simulink model "M10B39"  (R2025a)
settings: Solver=ode23tb  StartTime=0.0  StopTime=20  FixedStep=0.001  MaxStep=0.01  RelTol=1e-3  EnableMultiTasking=on
InitFcn:
  | initAll
values from neighbouring files (symbols this model uses):
  acom = 100    [initAll.m]    (also in initAll_V2.m)
  bcom = 50    [initAll.m]    (also in initAll_V2.m)
  commun = 0*commun    [initAll.m]    (also in initAll_V2.m)
  DataDelay = 0.0*DataDelay    [initAll.m]    (also in initAll_V2.m)
  fB = 50    [initAll.m]    (also in initAll_V2.m)
  Geninit = Generator_init(opdata,SynMach_in_gidx)    [initAll.m]    (also in initAll_V2.m)
  lam = 100    [initAll.m]    (also in initAll_V2.m)
  SgridB = 100    [initAll.m]    (also in initAll_V2.m)
  wB = 2*pi*fB    (= 314.159265359)    [initAll.m]    (also in initAll_V2.m)
undefined symbols (not defined in the file or in its folder): AVm0, c1, c2, c3, c4, c5, c6, cp_nom, ESinit, lambda_nom, P_wind_base, Pelec_base, Pnom, Windinit, YY_load
libraries: spsBistableLib x10, simulink_extras x6, simulink x1
(part 3 of 8)

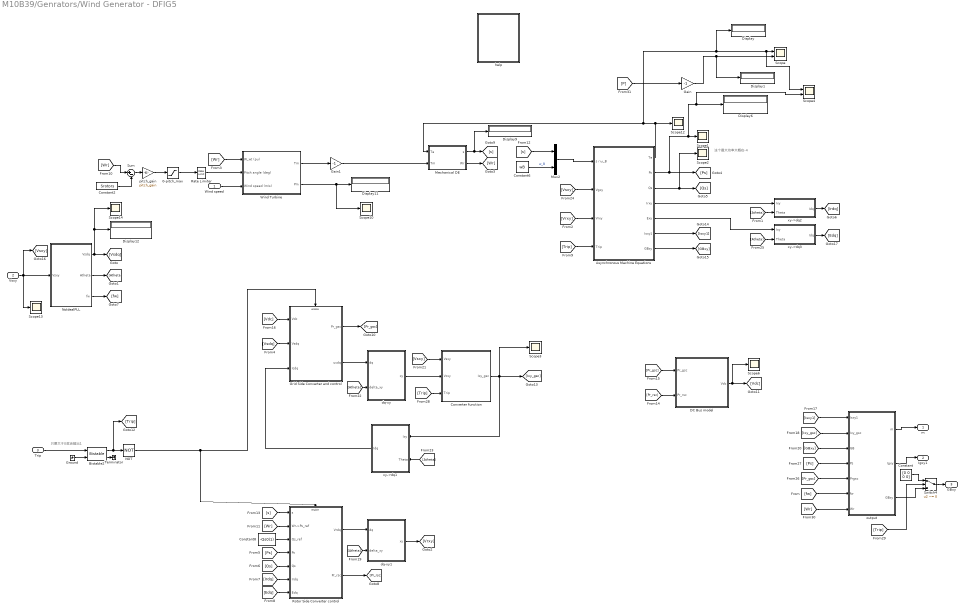
== system M10B39/Genrators/Wind Generator - DFIG5 ==
  note: 只要大于0就会输出1
  note: 这个最大功率大概在-4
  Wind speed : Inport
  Vsxy : Inport  Port=2
  Trip : Inport  Port=3
  0-pitch_max : Saturate  UpperLimit=pitch_max  LowerLimit=0
  "Asynchronous Machine Equations " : Subsystem
  Bistable2 : spsBistableLib/Bistable  Qpriority=Set  ic=0  Ts=0
  Constant : Constant  Value=[0 0 0 0]
  Constant2 : Constant  Value=Srotors
  Constant6 : Constant  Value=wB
  Constant8 : Constant  Value=-Qs0(1)
  Converter function : Subsystem
  DC Bus model : Subsystem
  Display{,1,6,9,11..12} (6 alike) : Display
  Gain : Gain  Gain=-1
  Gain1 : Gain  Gain=-1
  Grid Side Converter and control : Subsystem
  Ground : Ground
  Mechanical DE : Subsystem
  Mux2 : Mux  Inputs=2
  NOT : Logic  Operator=NOT  AllPortsSameDT=off  OutDataTypeStr=boolean
  NoIdealPLL : Subsystem  VariantControl=Noideal_PLL_Wind1
  "Rate Limiter   " : RateLimiter  RisingSlewLimit=pitch_rate  FallingSlewLimit=-pitch_rate
  Rotor Side Converter control : Subsystem
  Scope : Scope  NumInputPorts=2
      settings: ActiveDisplayYMinimum=-1.1471  ActiveDisplayYMaximum=-0.81376
  Scope{1..3,6,10,12..14} (8 alike) : Scope
      Scope1 settings: ActiveDisplayYMinimum=-2.187000000000014  ActiveDisplayYMaximum=-2.186999999999987  DataLoggingVariableName=ScopeData2
      Scope10 settings: ActiveDisplayYMinimum=0.84538  ActiveDisplayYMaximum=0.84729
      Scope12 settings: ActiveDisplayYMinimum=-1.99497  ActiveDisplayYMaximum=-0.90484  DataLoggingVariableName=ScopeData6
      Scope13 settings: ActiveDisplayYMinimum=-1.25875  ActiveDisplayYMaximum=1.25908  DataLoggingVariableName=ScopeData2
      Scope14 settings: ActiveDisplayYMinimum=1.003489  ActiveDisplayYMaximum=1.0035  DataLoggingVariableName=ScopeData3
      Scope2 settings: ActiveDisplayYMinimum=-0.00085  ActiveDisplayYMaximum=0.00099  DataLoggingVariableName=ScopeData2
      Scope3 settings: ActiveDisplayYMinimum=-0.01172  ActiveDisplayYMaximum=0.10551
      Scope6 settings: ActiveDisplayYMinimum=2.82799999999992  ActiveDisplayYMaximum=2.82800000000004  DataLoggingVariableName=ScopeData5
  Scope4 : Scope  NumInputPorts=2
      settings: ActiveDisplayYMinimum=-1.13533  ActiveDisplayYMaximum=-0.91965  DataLoggingVariableName=ScopeData2
  Sum : Sum  Inputs=|+-  SaturateOnIntegerOverflow=on
  Switch4 : Switch  Criteria=u2 ~= 0  Threshold=0.5  InputSameDT=off
  Terminator : Terminator
  Wind Turbine : Subsystem
  dq-xy : Subsystem
  dq-xy1 : Subsystem
  help : Subsystem
  output : Subsystem
  pitch_gain : Gain  Gain=pitch_gain  SaturateOnIntegerOverflow=on  OutDataTypeStr=Inherit: Same as input  ParamDataTypeStr=Inherit: Same as input
  xy->dq1 : Subsystem
  xy->dq2 : Subsystem
  xy->dq3 : Subsystem
  m : Outport
  Igxy1 : Outport  Port=2
  GBxy : Outport  Port=3
  wires:
  [Wr] -> output/7(Wr)
  Gain1/1 -> Mechanical DE/2(Tm)
  output/3(GBxy) -> Switch4/3
  Switch4/1 -> GBxy/1
  Constant/1 -> Switch4/1
  [Trip] -> Switch4/2
  [Trip] -> Converter function/3(Trip)
  [Trip] -> "Asynchronous Machine Equations "/4("Trip ")
  [Wr] -> Sum/1
  0-pitch_max/1 -> "Rate Limiter   "/1
  pitch_gain/1 -> 0-pitch_max/1
  Constant2/1 -> Sum/2
  Sum/1 -> pitch_gain/1
  NOT/1 -> Rotor Side Converter control/Enable, Grid Side Converter and control/Enable
  Trip/1 -> Bistable2/1
  Bistable2/2 -> Terminator/1
  Bistable2/1 -> NOT/1, [Trip]
  Ground/1 -> Bistable2/2
  [fw] -> output/6(fw)
  [Pr_gsc] -> output/5(Prgsc)
  [Ps] -> output/4(Ps)
  output/1(m) -> m/1
  [Isxy1] -> output/1(Isxy1)
  [Ixy_gsc] -> output/2(Ixy_gsc)
  output/2(Igxy) -> Igxy1/1
  xy->dq3/1(Idq) -> [Edq]
  [Atheta] -> xy->dq3/2(Theta)
  xy->dq2/1(Idq) -> [Irdq]
  [Atheta] -> xy->dq2/2(Theta)
  dq-xy1/1(xy) -> [Vrxy]
  [Atheta] -> dq-xy1/2(delta_xy)
  xy->dq1/1(Idq) -> Grid Side Converter and control/3(Icdq)
  [Atheta] -> xy->dq1/2(Theta)
  [Atheta] -> dq-xy/2(delta_xy)
  dq-xy/1(xy) -> Converter function/2(Vcxy)
  Grid Side Converter and control/2(ucdq) -> dq-xy/1(dq)
  [Vsxy] -> Converter function/1(Vsxy)
  NoIdealPLL/3(fw) -> [fw]
  Vsxy/1 -> [Vsxy], Scope13/1, NoIdealPLL/1(Vsxy)
  [GBxy] -> output/3(GB)
  [Pr_rsc] -> DC Bus model/2(Pr_rsc)
  "Asynchronous Machine Equations "/1(Te) -> Scope12/1, Display/1, Scope4/1, Scope/1, Mechanical DE/1(Te)
  Constant8/1 -> Rotor Side Converter control/3(Qs_ref)
  [Wr] -> Wind Turbine/1(W_wt (pu))
  "Asynchronous Machine Equations "/4(Irxy) -> xy->dq2/1(Ixy)
  Converter function/1(Ixy_gsc) -> [Ixy_gsc], xy->dq1/1(Ixy), Scope3/1
  [Vrxy] -> "Asynchronous Machine Equations "/3(Vrxy)
  "Asynchronous Machine Equations "/6(Isxy1) -> [Isxy1]
  [Qs] -> Rotor Side Converter control/5(Qs)
  [Vdc] -> Grid Side Converter and control/1(Vdc)
  [Pr_gsc] -> DC Bus model/1(Pr_gsc)
  "Asynchronous Machine Equations "/2(Ps) -> Scope1/1, Scope4/2, Display6/1, [Ps]
  Mechanical DE/1("s ") -> [s], Display9/1
  [s] -> Mux2/1
  [Vsdq] -> Grid Side Converter and control/2(Vsdq)
  Grid Side Converter and control/1(Pr_gsc) -> [Pr_gsc]
  NoIdealPLL/2(Atheta) -> [Atheta]
  DC Bus model/1(Vdc) -> [Vdc], Scope6/1
  [Vsxy] -> "Asynchronous Machine Equations "/2(Vgxy)
  Wind Turbine/1(Tm) -> Gain1/1
  [Irdq] -> Rotor Side Converter control/6(Irdq)
  Mux2/1 -> "Asynchronous Machine Equations "/1(s / ω_B)
  "Asynchronous Machine Equations "/7(GBxy) -> [GBxy]
  "Rate Limiter   "/1 -> Wind Turbine/2(Pitch angle (deg))
  NoIdealPLL/1(Vsdq) -> Display12/1, Scope14/1, [Vsdq]
  [s] -> Rotor Side Converter control/1(s)
  Rotor Side Converter control/2(Pr_rsc) -> [Pr_rsc]
  Mechanical DE/2(Wr) -> [Wr]
  [Wr] -> Rotor Side Converter control/2(Wr->Ps_ref)
  Wind Turbine/2(Pm) -> Display11/1, Scope10/1
  "Asynchronous Machine Equations "/3(Qs) -> [Qs], Scope2/1
  Wind speed/1 -> Wind Turbine/3(Wind speed (m/s))
  [Ps] -> Rotor Side Converter control/4(Ps)
  Rotor Side Converter control/1(Vrdq) -> dq-xy1/1(dq)
  [Edq] -> Rotor Side Converter control/7(Edq)
  Constant6/1 -> Mux2/2  "w_B"
  "Asynchronous Machine Equations "/5(Exy) -> xy->dq3/1(Ixy)
  [P] -> Gain/1
  Gain/1 -> Display1/1, Scope/2

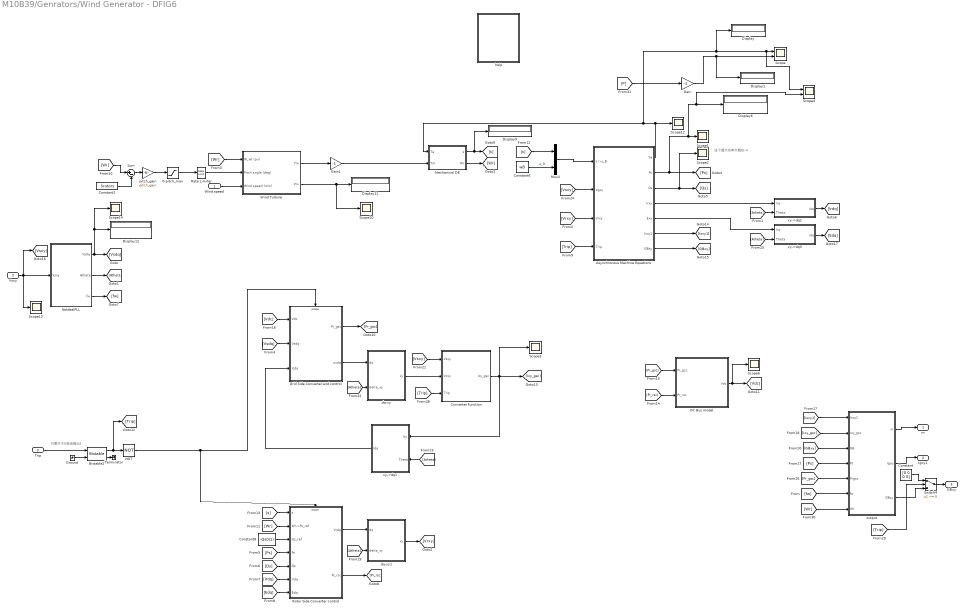
== system M10B39/Genrators/Wind Generator - DFIG6 ==
  note: 只要大于0就会输出1
  note: 这个最大功率大概在-4
  Wind speed : Inport
  Vsxy : Inport  Port=2
  Trip : Inport  Port=3
  0-pitch_max : Saturate  UpperLimit=pitch_max  LowerLimit=0
  "Asynchronous Machine Equations " : Subsystem
  Bistable2 : spsBistableLib/Bistable  Qpriority=Set  ic=0  Ts=0
  Constant : Constant  Value=[0 0 0 0]
  Constant2 : Constant  Value=Srotors
  Constant6 : Constant  Value=wB
  Constant8 : Constant  Value=-Qs0(1)
  Converter function : Subsystem
  DC Bus model : Subsystem
  Display{,1,6,9,11..12} (6 alike) : Display
  Gain : Gain  Gain=-1
  Gain1 : Gain  Gain=-1
  Grid Side Converter and control : Subsystem
  Ground : Ground
  Mechanical DE : Subsystem
  Mux2 : Mux  Inputs=2
  NOT : Logic  Operator=NOT  AllPortsSameDT=off  OutDataTypeStr=boolean
  NoIdealPLL : Subsystem  VariantControl=Noideal_PLL_Wind1
  "Rate Limiter   " : RateLimiter  RisingSlewLimit=pitch_rate  FallingSlewLimit=-pitch_rate
  Rotor Side Converter control : Subsystem
  Scope : Scope  NumInputPorts=2
      settings: ActiveDisplayYMinimum=-1.1471  ActiveDisplayYMaximum=-0.81376
  Scope{1..3,6,10,12..14} (8 alike) : Scope
      Scope1 settings: ActiveDisplayYMinimum=-2.187000000000014  ActiveDisplayYMaximum=-2.186999999999987  DataLoggingVariableName=ScopeData2
      Scope10 settings: ActiveDisplayYMinimum=0.84538  ActiveDisplayYMaximum=0.84729
      Scope12 settings: ActiveDisplayYMinimum=-1.99497  ActiveDisplayYMaximum=-0.90484  DataLoggingVariableName=ScopeData6
      Scope13 settings: ActiveDisplayYMinimum=-1.25875  ActiveDisplayYMaximum=1.25908  DataLoggingVariableName=ScopeData2
      Scope14 settings: ActiveDisplayYMinimum=1.003489  ActiveDisplayYMaximum=1.0035  DataLoggingVariableName=ScopeData3
      Scope2 settings: ActiveDisplayYMinimum=-0.00085  ActiveDisplayYMaximum=0.00099  DataLoggingVariableName=ScopeData2
      Scope3 settings: ActiveDisplayYMinimum=-0.01172  ActiveDisplayYMaximum=0.10551
      Scope6 settings: ActiveDisplayYMinimum=2.82799999999992  ActiveDisplayYMaximum=2.82800000000004  DataLoggingVariableName=ScopeData5
  Scope4 : Scope  NumInputPorts=2
      settings: ActiveDisplayYMinimum=-1.13533  ActiveDisplayYMaximum=-0.91965  DataLoggingVariableName=ScopeData2
  Sum : Sum  Inputs=|+-  SaturateOnIntegerOverflow=on
  Switch4 : Switch  Criteria=u2 ~= 0  Threshold=0.5  InputSameDT=off
  Terminator : Terminator
  Wind Turbine : Subsystem
  dq-xy : Subsystem
  dq-xy1 : Subsystem
  help : Subsystem
  output : Subsystem
  pitch_gain : Gain  Gain=pitch_gain  SaturateOnIntegerOverflow=on  OutDataTypeStr=Inherit: Same as input  ParamDataTypeStr=Inherit: Same as input
  xy->dq1 : Subsystem
  xy->dq2 : Subsystem
  xy->dq3 : Subsystem
  m : Outport
  Igxy1 : Outport  Port=2
  GBxy : Outport  Port=3
  wires:
  [Wr] -> output/7(Wr)
  Gain1/1 -> Mechanical DE/2(Tm)
  output/3(GBxy) -> Switch4/3
  Switch4/1 -> GBxy/1
  Constant/1 -> Switch4/1
  [Trip] -> Switch4/2
  [Trip] -> Converter function/3(Trip)
  [Trip] -> "Asynchronous Machine Equations "/4("Trip ")
  [Wr] -> Sum/1
  0-pitch_max/1 -> "Rate Limiter   "/1
  pitch_gain/1 -> 0-pitch_max/1
  Constant2/1 -> Sum/2
  Sum/1 -> pitch_gain/1
  NOT/1 -> Rotor Side Converter control/Enable, Grid Side Converter and control/Enable
  Trip/1 -> Bistable2/1
  Bistable2/2 -> Terminator/1
  Bistable2/1 -> NOT/1, [Trip]
  Ground/1 -> Bistable2/2
  [fw] -> output/6(fw)
  [Pr_gsc] -> output/5(Prgsc)
  [Ps] -> output/4(Ps)
  output/1(m) -> m/1
  [Isxy1] -> output/1(Isxy1)
  [Ixy_gsc] -> output/2(Ixy_gsc)
  output/2(Igxy) -> Igxy1/1
  xy->dq3/1(Idq) -> [Edq]
  [Atheta] -> xy->dq3/2(Theta)
  xy->dq2/1(Idq) -> [Irdq]
  [Atheta] -> xy->dq2/2(Theta)
  dq-xy1/1(xy) -> [Vrxy]
  [Atheta] -> dq-xy1/2(delta_xy)
  xy->dq1/1(Idq) -> Grid Side Converter and control/3(Icdq)
  [Atheta] -> xy->dq1/2(Theta)
  [Atheta] -> dq-xy/2(delta_xy)
  dq-xy/1(xy) -> Converter function/2(Vcxy)
  Grid Side Converter and control/2(ucdq) -> dq-xy/1(dq)
  [Vsxy] -> Converter function/1(Vsxy)
  NoIdealPLL/3(fw) -> [fw]
  Vsxy/1 -> [Vsxy], Scope13/1, NoIdealPLL/1(Vsxy)
  [GBxy] -> output/3(GB)
  [Pr_rsc] -> DC Bus model/2(Pr_rsc)
  "Asynchronous Machine Equations "/1(Te) -> Scope12/1, Display/1, Scope4/1, Scope/1, Mechanical DE/1(Te)
  Constant8/1 -> Rotor Side Converter control/3(Qs_ref)
  [Wr] -> Wind Turbine/1(W_wt (pu))
  "Asynchronous Machine Equations "/4(Irxy) -> xy->dq2/1(Ixy)
  Converter function/1(Ixy_gsc) -> [Ixy_gsc], xy->dq1/1(Ixy), Scope3/1
  [Vrxy] -> "Asynchronous Machine Equations "/3(Vrxy)
  "Asynchronous Machine Equations "/6(Isxy1) -> [Isxy1]
  [Qs] -> Rotor Side Converter control/5(Qs)
  [Vdc] -> Grid Side Converter and control/1(Vdc)
  [Pr_gsc] -> DC Bus model/1(Pr_gsc)
  "Asynchronous Machine Equations "/2(Ps) -> Scope1/1, Scope4/2, Display6/1, [Ps]
  Mechanical DE/1("s ") -> [s], Display9/1
  [s] -> Mux2/1
  [Vsdq] -> Grid Side Converter and control/2(Vsdq)
  Grid Side Converter and control/1(Pr_gsc) -> [Pr_gsc]
  NoIdealPLL/2(Atheta) -> [Atheta]
  DC Bus model/1(Vdc) -> [Vdc], Scope6/1
  [Vsxy] -> "Asynchronous Machine Equations "/2(Vgxy)
  Wind Turbine/1(Tm) -> Gain1/1
  [Irdq] -> Rotor Side Converter control/6(Irdq)
  Mux2/1 -> "Asynchronous Machine Equations "/1(s / ω_B)
  "Asynchronous Machine Equations "/7(GBxy) -> [GBxy]
  "Rate Limiter   "/1 -> Wind Turbine/2(Pitch angle (deg))
  NoIdealPLL/1(Vsdq) -> Display12/1, Scope14/1, [Vsdq]
  [s] -> Rotor Side Converter control/1(s)
  Rotor Side Converter control/2(Pr_rsc) -> [Pr_rsc]
  Mechanical DE/2(Wr) -> [Wr]
  [Wr] -> Rotor Side Converter control/2(Wr->Ps_ref)
  Wind Turbine/2(Pm) -> Display11/1, Scope10/1
  "Asynchronous Machine Equations "/3(Qs) -> [Qs], Scope2/1
  Wind speed/1 -> Wind Turbine/3(Wind speed (m/s))
  [Ps] -> Rotor Side Converter control/4(Ps)
  Rotor Side Converter control/1(Vrdq) -> dq-xy1/1(dq)
  [Edq] -> Rotor Side Converter control/7(Edq)
  Constant6/1 -> Mux2/2  "w_B"
  "Asynchronous Machine Equations "/5(Exy) -> xy->dq3/1(Ixy)
  [P] -> Gain/1
  Gain/1 -> Display1/1, Scope/2

== system M10B39/Genrators/ES1/ control1 ==
  usdq : Inport
  isdq : Inport  Port=2
  delta : Inport  Port=3
  Enable : EnablePort
  Add : Sum  Inputs=|-+
  Add2 : Sum  Inputs=|-+
  Add3 : Sum
  Add4 : Sum  Inputs=-+
  Add6 : Sum  Inputs=|++
  Add7 : Sum  Inputs=+-
  Complex to Magnitude-Angle : ComplexToMagnitudeAngle
  Complex to Real-Imag1 : ComplexToRealImag
  Constant : Constant
  Constant1 : Constant  Value=usd0
  Constant2 : Constant  Value=0
  Constant3 : Constant  Value=Q0
  Constant4 : Constant
  Demux : Demux  Outputs=2
  Demux1 : Demux  Outputs=2
  Gain : Gain  Gain=0.01
  Gain1 : Gain  Gain=-1
  K5 : Gain  Gain=Lpr  SaturateOnIntegerOverflow=on  OutDataTypeStr=Inherit: Same as input  ParamDataTypeStr=Inherit: Same as input
  K6 : Gain  Gain=Lpr  SaturateOnIntegerOverflow=on  OutDataTypeStr=Inherit: Same as input  ParamDataTypeStr=Inherit: Same as input
  Magnitude-Angle to Complex : MagnitudeAngleToComplex
  Product{1,4..6} (4 alike) : Product  RndMeth=Zero
  Real-Imag to Complex : RealImagToComplex
  Scope : Scope
      settings: ActiveDisplayYMinimum=-1.90229  ActiveDisplayYMaximum=-1.00495  DataLoggingVariableName=ScopeData6
  Scope1 : Scope
      settings: ActiveDisplayYMinimum=1.01143  ActiveDisplayYMaximum=1.18506  DataLoggingVariableName=ScopeData8
  Scope2 : Scope  NumInputPorts=2
      settings: ActiveDisplayYMinimum=-1E-15  ActiveDisplayYMaximum=1.3E-14  DataLoggingVariableName=ScopeData9
  Scope3 : Scope  NumInputPorts=2
      settings: ActiveDisplayYMinimum=-0.06902  ActiveDisplayYMaximum=1.69489  DataLoggingVariableName=ScopeData4
  Scope7 : Scope  NumInputPorts=2
      settings: ActiveDisplayYMinimum=-1.01296  ActiveDisplayYMaximum=-0.62415
  Sum : Sum  Inputs=|+-
  Sum2 : Sum  Inputs=|+-  SaturateOnIntegerOverflow=on
  Sum23 : Sum  Inputs=|+-  SaturateOnIntegerOverflow=on
  Sum9 : Sum  Inputs=|+-  SaturateOnIntegerOverflow=on
  control_AC_voltage : Subsystem  VariantControl=VSC1q_Variant2
  control_AC_voltage1 : Subsystem  VariantControl=VSC1q_Variant2
  in_D_PI : Subsystem  mask{KP_=KpId_VSC_A, KI_=KiId_VSC_A, Upper_limit=inf, Lower_limit=-inf, Upper_saturation_limit=inf, Lower_saturation_limit=-inf, integrator_init=Md_A_0}
      mask prompts: KP_ "比例系数P"; KI_ "积分系数I"; Upper_limit "限幅上限"; Lower_limit "限幅下限"; Upper_saturation_limit "积分饱和上限"; Lower_saturation_limit "积分饱和下限"; integrator_init "积分初始值"
      mask DialogControl Container4 Prompt: 控制参数
      mask DialogControl Container5 Prompt: 初始值
      mask Display: disp('PI')
  in_Q_PI : Subsystem  mask{KP_=KpIq_VSC_A, KI_=KiIq_VSC_A, Upper_limit=inf, Lower_limit=-inf, Upper_saturation_limit=inf, Lower_saturation_limit=-inf, integrator_init=Mq_A_0}
      mask prompts: KP_ "比例系数P"; KI_ "积分系数I"; Upper_limit "限幅上限"; Lower_limit "限幅下限"; Upper_saturation_limit "积分饱和上限"; Lower_saturation_limit "积分饱和下限"; integrator_init "积分初始值"
      mask DialogControl Container4 Prompt: 控制参数
      mask DialogControl Container5 Prompt: 初始值
      mask Display: disp('PI')
  ucx : Outport
  ucy : Outport  Port=2
  wires:
  Magnitude-Angle to Complex/1 -> Complex to Real-Imag1/1
  Add/1 -> Real-Imag to Complex/2
  Add2/1 -> Real-Imag to Complex/1
  delta/1 -> Add6/2
  Add6/1 -> Magnitude-Angle to Complex/2
  Complex to Magnitude-Angle/2 -> Add6/1
  Sum9/1 -> in_D_PI/1(In1)
  K5/1 -> Add3/1
  [usd] -> Add3/2
  Add3/1 -> Add2/2
  in_D_PI/1(Out1) -> Add2/1
  Constant/1 -> Product4/2
  [isq] -> Product4/1
  [isd] -> Scope7/2, Sum9/2
  Product4/1 -> K5/1
  Demux1/1 -> [isd]
  Demux/1 -> [usd]
  Demux1/2 -> [isq]
  Demux/2 -> [usq]
  isdq/1 -> Demux1/1
  usdq/1 -> Demux/1
  [usq] -> Add4/2
  K6/1 -> Add4/1
  in_Q_PI/1(Out1) -> Add/1
  Sum23/1 -> in_Q_PI/1(In1)
  [isd] -> Product1/1
  [isq] -> Sum23/2, Scope3/2
  Product1/1 -> K6/1
  Constant4/1 -> Product1/2
  Add4/1 -> Add/2
  Real-Imag to Complex/1 -> Complex to Magnitude-Angle/1
  Complex to Magnitude-Angle/1 -> Magnitude-Angle to Complex/1
  Complex to Real-Imag1/1 -> ucx/1
  Complex to Real-Imag1/2 -> ucy/1
  [usd] -> Scope1/1, control_AC_voltage/1(usd)
  control_AC_voltage/1(isdref) -> Scope7/1, Sum9/1
  [isq] -> Product5/2
  Product5/1 -> Add7/2
  [usd] -> Product5/1
  [isd] -> Product6/2
  Product6/1 -> Add7/1
  [usq] -> Product6/1
  Gain/1 -> Sum/2
  control_AC_voltage1/1(isqref) -> Scope3/1, Sum23/1
  [usq] -> Scope2/1, control_AC_voltage1/1(usq)
  Constant2/1 -> Scope2/2, control_AC_voltage1/2(usqref)
  Add7/1 -> Scope/1, Gain1/1
  Sum2/1 -> Gain/1
  Constant3/1 -> Sum2/2
  Gain1/1 -> Sum2/1
  Sum/1 -> control_AC_voltage/2(usdref)
  Constant1/1 -> Sum/1

== system M10B39/Genrators/ES1/in_D_PI ==
  In1 : Inport
  Ki : Gain  Gain=KI_  SaturateOnIntegerOverflow=on  OutDataTypeStr=Inherit: Same as input  ParamDataTypeStr=Inherit: Same as input
  Kp : Gain  Gain=KP_  SaturateOnIntegerOverflow=on  OutDataTypeStr=Inherit: Same as input  ParamDataTypeStr=Inherit: Same as input
  Saturation2 : Saturate  UpperLimit=Upper_limit  LowerLimit=Lower_limit
  Sum12 : Sum  SaturateOnIntegerOverflow=on
  integrator : Integrator  InitialCondition=integrator_init  LimitOutput=on  UpperSaturationLimit=Upper_saturation_limit  LowerSaturationLimit=Lower_saturation_limit
  Out1 : Outport
  wires:
  In1/1 -> Ki/1, Kp/1
  Kp/1 -> Sum12/2
  Ki/1 -> integrator/1
  integrator/1 -> Sum12/1
  Saturation2/1 -> Out1/1
  Sum12/1 -> Saturation2/1

== system M10B39/Genrators/ES1/output ==
  is_xy : Inport
  Pe : Inport  Port=2
  Brecx : Constant  Value=0
  Brecy : Constant  Value=0
  Bus Creator : BusCreator  Inputs=4
  Constant : Constant
  Gain : Gain  Gain=SvscB./SgridB
  Gain1 : Gain  Gain=-1
  Gain2 : Gain  Gain=-1
  Gain6 : Gain
  Grecx : Constant  Value=0
  Grecy : Constant  Value=0
  Mux3 : Mux
  Sum : Sum  Inputs=|++
  m : Outport
  isxy : Outport  Port=2
  GBxy : Outport  Port=3
  wires:
  Bus Creator/1 -> m/1
  Gain6/1 -> GBxy/1, Bus Creator/4  "GBxy"
  Mux3/1 -> Gain6/1
  Grecx/1 -> Mux3/1
  Brecx/1 -> Mux3/3
  Grecy/1 -> Mux3/2
  Brecy/1 -> Mux3/4
  Gain1/1 -> isxy/1, Bus Creator/1  "is_xy"
  Gain2/1 -> Bus Creator/2  "Pe"
  Gain/1 -> Gain1/1  "is_xy"
  Pe/1 -> Gain2/1  "Pe"
  [WreES1] -> Sum/1  "Pe"
  Constant/1 -> Sum/2
  Sum/1 -> Bus Creator/3  "w"
  is_xy/1 -> Gain/1

== system M10B39/Genrators/ES1/xy->dq ==
  Ixy : Inport
  Theta : Inport  Port=2
  Complex to Magnitude-Angle : ComplexToMagnitudeAngle
  Complex to Real-Imag : ComplexToRealImag
  Demux1 : Demux  Outputs=2
      settings: DisplayOption=none
  Magnitude-Angle to Complex : MagnitudeAngleToComplex
  Mux : Mux  Inputs=2
  Real-Imag to Complex : RealImagToComplex
  Scope : Scope
      settings: ActiveDisplayYMinimum=3.11918  ActiveDisplayYMaximum=3.16079
  Scope1 : Scope
      settings: ActiveDisplayYMinimum=2.59405  ActiveDisplayYMaximum=3.13201  DataLoggingVariableName=ScopeData3
  Sum1 : Sum  Inputs=|+-  SaturateOnIntegerOverflow=on
  Idq : Outport
  wires:
  Complex to Magnitude-Angle/1 -> Magnitude-Angle to Complex/1
  Theta/1 -> Sum1/2
  Complex to Magnitude-Angle/2 -> Sum1/1, Scope1/1
  Demux1/1 -> Real-Imag to Complex/1
  Complex to Real-Imag/2 -> Mux/2  "Iq"
  Mux/1 -> Idq/1
  Complex to Real-Imag/1 -> Mux/1  "Id"
  Magnitude-Angle to Complex/1 -> Complex to Real-Imag/1
  Sum1/1 -> Magnitude-Angle to Complex/2, Scope/1
  Demux1/2 -> Real-Imag to Complex/2
  Real-Imag to Complex/1 -> Complex to Magnitude-Angle/1
  Ixy/1 -> Demux1/1

== system M10B39/Genrators/ES2/ control1 ==
  usdq : Inport
  isdq : Inport  Port=2
  delta : Inport  Port=3
  Enable : EnablePort
  Add : Sum  Inputs=|-+
  Add2 : Sum  Inputs=|-+
  Add3 : Sum
  Add4 : Sum  Inputs=-+
  Add6 : Sum  Inputs=|++
  Add7 : Sum  Inputs=+-
  Complex to Magnitude-Angle : ComplexToMagnitudeAngle
  Complex to Real-Imag1 : ComplexToRealImag
  Constant : Constant
  Constant1 : Constant  Value=usd0
  Constant2 : Constant  Value=0
  Constant3 : Constant  Value=Q0
  Constant4 : Constant
  Demux : Demux  Outputs=2
  Demux1 : Demux  Outputs=2
  Gain : Gain  Gain=0.01
  Gain1 : Gain  Gain=-1
  K5 : Gain  Gain=Lpr  SaturateOnIntegerOverflow=on  OutDataTypeStr=Inherit: Same as input  ParamDataTypeStr=Inherit: Same as input
  K6 : Gain  Gain=Lpr  SaturateOnIntegerOverflow=on  OutDataTypeStr=Inherit: Same as input  ParamDataTypeStr=Inherit: Same as input
  Magnitude-Angle to Complex : MagnitudeAngleToComplex
  Product{1,4..6} (4 alike) : Product  RndMeth=Zero
  Real-Imag to Complex : RealImagToComplex
  Scope{,1..2,7} (4 alike) : Scope
      Scope settings: ActiveDisplayYMinimum=-2.62202  ActiveDisplayYMaximum=-0.62202  DataLoggingVariableName=ScopeData6
      Scope1 settings: ActiveDisplayYMinimum=0.03  ActiveDisplayYMaximum=2.03  DataLoggingVariableName=ScopeData8
      Scope2 settings: ActiveDisplayYMinimum=-1.2875  ActiveDisplayYMaximum=1.2875  DataLoggingVariableName=ScopeData9
      Scope7 settings: ActiveDisplayYMinimum=-7.47817  ActiveDisplayYMaximum=-5.47817
  Sum : Sum  Inputs=|+-
  Sum2 : Sum  Inputs=|+-  SaturateOnIntegerOverflow=on
  Sum23 : Sum  Inputs=|+-  SaturateOnIntegerOverflow=on
  Sum9 : Sum  Inputs=|+-  SaturateOnIntegerOverflow=on
  control_AC_voltage : Subsystem  VariantControl=VSC1q_Variant2
  control_AC_voltage1 : Subsystem  VariantControl=VSC1q_Variant2
  in_D_PI : Subsystem  mask{KP_=KpId_VSC_A, KI_=KiId_VSC_A, Upper_limit=inf, Lower_limit=-inf, Upper_saturation_limit=inf, Lower_saturation_limit=-inf, integrator_init=Md_A_0}
      mask prompts: KP_ "比例系数P"; KI_ "积分系数I"; Upper_limit "限幅上限"; Lower_limit "限幅下限"; Upper_saturation_limit "积分饱和上限"; Lower_saturation_limit "积分饱和下限"; integrator_init "积分初始值"
      mask DialogControl Container4 Prompt: 控制参数
      mask DialogControl Container5 Prompt: 初始值
      mask Display: disp('PI')
  in_Q_PI : Subsystem  mask{KP_=KpIq_VSC_A, KI_=KiIq_VSC_A, Upper_limit=inf, Lower_limit=-inf, Upper_saturation_limit=inf, Lower_saturation_limit=-inf, integrator_init=Mq_A_0}
      mask prompts: KP_ "比例系数P"; KI_ "积分系数I"; Upper_limit "限幅上限"; Lower_limit "限幅下限"; Upper_saturation_limit "积分饱和上限"; Lower_saturation_limit "积分饱和下限"; integrator_init "积分初始值"
      mask DialogControl Container4 Prompt: 控制参数
      mask DialogControl Container5 Prompt: 初始值
      mask Display: disp('PI')
  ucx : Outport
  ucy : Outport  Port=2
  wires:
  Magnitude-Angle to Complex/1 -> Complex to Real-Imag1/1
  Add/1 -> Real-Imag to Complex/2
  Add2/1 -> Real-Imag to Complex/1
  delta/1 -> Add6/2
  Add6/1 -> Magnitude-Angle to Complex/2
  Complex to Magnitude-Angle/2 -> Add6/1
  Sum9/1 -> in_D_PI/1(In1)
  K5/1 -> Add3/1
  [usd] -> Add3/2
  Add3/1 -> Add2/2
  in_D_PI/1(Out1) -> Add2/1
  Constant/1 -> Product4/2
  [isq] -> Product4/1
  [isd] -> Sum9/2
  Product4/1 -> K5/1
  Demux1/1 -> [isd]
  Demux/1 -> [usd]
  Demux1/2 -> [isq]
  Demux/2 -> [usq]
  isdq/1 -> Demux1/1
  usdq/1 -> Demux/1
  [usq] -> Add4/2
  K6/1 -> Add4/1
  in_Q_PI/1(Out1) -> Add/1
  Sum23/1 -> in_Q_PI/1(In1)
  [isd] -> Product1/1
  [isq] -> Sum23/2
  Product1/1 -> K6/1
  Constant4/1 -> Product1/2
  Add4/1 -> Add/2
  Real-Imag to Complex/1 -> Complex to Magnitude-Angle/1
  Complex to Magnitude-Angle/1 -> Magnitude-Angle to Complex/1
  Complex to Real-Imag1/1 -> ucx/1
  Complex to Real-Imag1/2 -> ucy/1
  [usd] -> Scope1/1, control_AC_voltage/1(usd)
  control_AC_voltage/1(isdref) -> Scope7/1, Sum9/1
  [isq] -> Product5/2
  Product5/1 -> Add7/2
  [usd] -> Product5/1
  [isd] -> Product6/2
  Product6/1 -> Add7/1
  [usq] -> Product6/1
  Gain/1 -> Sum/2
  control_AC_voltage1/1(isqref) -> Sum23/1
  [usq] -> Scope2/1, control_AC_voltage1/1(usq)
  Constant2/1 -> control_AC_voltage1/2(usqref)
  Add7/1 -> Scope/1, Gain1/1
  Sum2/1 -> Gain/1
  Constant3/1 -> Sum2/2
  Gain1/1 -> Sum2/1
  Sum/1 -> control_AC_voltage/2(usdref)
  Constant1/1 -> Sum/1

== system M10B39/Genrators/ES2/output ==
  is_xy : Inport
  Pe : Inport  Port=2
  Brecx : Constant  Value=0
  Brecy : Constant  Value=0
  Bus Creator : BusCreator  Inputs=4
  Constant : Constant
  Gain : Gain  Gain=SvscB./SgridB
  Gain1 : Gain  Gain=-1
  Gain2 : Gain  Gain=-1
  Gain6 : Gain
  Grecx : Constant  Value=0
  Grecy : Constant  Value=0
  Mux3 : Mux
  Sum : Sum  Inputs=|++
  m : Outport
  isxy : Outport  Port=2
  GBxy : Outport  Port=3
  wires:
  Bus Creator/1 -> m/1
  Gain6/1 -> GBxy/1, Bus Creator/4  "GBxy"
  Mux3/1 -> Gain6/1
  Grecx/1 -> Mux3/1
  Brecx/1 -> Mux3/3
  Grecy/1 -> Mux3/2
  Brecy/1 -> Mux3/4
  Gain1/1 -> isxy/1, Bus Creator/1  "is_xy"
  Gain2/1 -> Bus Creator/2  "Pe"
  Gain/1 -> Gain1/1  "is_xy"
  Pe/1 -> Gain2/1  "Pe"
  Constant/1 -> Sum/2
  [WreES2] -> Sum/1  "Pe"
  Sum/1 -> Bus Creator/3  "w"
  is_xy/1 -> Gain/1

== system M10B39/Genrators/ES2/xy->dq ==
  Ixy : Inport
  Theta : Inport  Port=2
  Complex to Magnitude-Angle : ComplexToMagnitudeAngle
  Complex to Real-Imag : ComplexToRealImag
  Demux1 : Demux  Outputs=2
      settings: DisplayOption=none
  Magnitude-Angle to Complex : MagnitudeAngleToComplex
  Mux : Mux  Inputs=2
  Real-Imag to Complex : RealImagToComplex
  Scope : Scope
      settings: ActiveDisplayYMinimum=3.11918  ActiveDisplayYMaximum=3.16079
  Scope1 : Scope
      settings: ActiveDisplayYMinimum=2.59405  ActiveDisplayYMaximum=3.13201  DataLoggingVariableName=ScopeData3
  Sum1 : Sum  Inputs=|+-  SaturateOnIntegerOverflow=on
  Idq : Outport
  wires:
  Complex to Magnitude-Angle/1 -> Magnitude-Angle to Complex/1
  Theta/1 -> Sum1/2
  Complex to Magnitude-Angle/2 -> Sum1/1, Scope1/1
  Demux1/1 -> Real-Imag to Complex/1
  Complex to Real-Imag/2 -> Mux/2  "Iq"
  Mux/1 -> Idq/1
  Complex to Real-Imag/1 -> Mux/1  "Id"
  Magnitude-Angle to Complex/1 -> Complex to Real-Imag/1
  Sum1/1 -> Magnitude-Angle to Complex/2, Scope/1
  Demux1/2 -> Real-Imag to Complex/2
  Real-Imag to Complex/1 -> Complex to Magnitude-Angle/1
  Ixy/1 -> Demux1/1

== system M10B39/Genrators/ES3/ control1 ==
  usdq : Inport
  isdq : Inport  Port=2
  delta : Inport  Port=3
  Enable : EnablePort
  Add : Sum  Inputs=|-+
  Add2 : Sum  Inputs=|-+
  Add3 : Sum
  Add4 : Sum  Inputs=-+
  Add6 : Sum  Inputs=|++
  Add7 : Sum  Inputs=+-
  Complex to Magnitude-Angle : ComplexToMagnitudeAngle
  Complex to Real-Imag1 : ComplexToRealImag
  Constant : Constant
  Constant1 : Constant  Value=usd0
  Constant2 : Constant  Value=0
  Constant3 : Constant  Value=Q0
  Constant4 : Constant
  Demux : Demux  Outputs=2
  Demux1 : Demux  Outputs=2
  Gain : Gain  Gain=0.01
  Gain1 : Gain  Gain=-1
  K5 : Gain  Gain=Lpr  SaturateOnIntegerOverflow=on  OutDataTypeStr=Inherit: Same as input  ParamDataTypeStr=Inherit: Same as input
  K6 : Gain  Gain=Lpr  SaturateOnIntegerOverflow=on  OutDataTypeStr=Inherit: Same as input  ParamDataTypeStr=Inherit: Same as input
  Magnitude-Angle to Complex : MagnitudeAngleToComplex
  Product{1,4..6} (4 alike) : Product  RndMeth=Zero
  Real-Imag to Complex : RealImagToComplex
  Scope{,1..2,7} (4 alike) : Scope
      Scope settings: ActiveDisplayYMinimum=-2.62202  ActiveDisplayYMaximum=-0.62202  DataLoggingVariableName=ScopeData6
      Scope1 settings: ActiveDisplayYMinimum=0.03  ActiveDisplayYMaximum=2.03  DataLoggingVariableName=ScopeData8
      Scope2 settings: ActiveDisplayYMinimum=-1.2875  ActiveDisplayYMaximum=1.2875  DataLoggingVariableName=ScopeData9
      Scope7 settings: ActiveDisplayYMinimum=-7.47817  ActiveDisplayYMaximum=-5.47817
  Sum : Sum  Inputs=|+-
  Sum2 : Sum  Inputs=|+-  SaturateOnIntegerOverflow=on
  Sum23 : Sum  Inputs=|+-  SaturateOnIntegerOverflow=on
  Sum9 : Sum  Inputs=|+-  SaturateOnIntegerOverflow=on
  control_AC_voltage : Subsystem  VariantControl=VSC1q_Variant2
  control_AC_voltage1 : Subsystem  VariantControl=VSC1q_Variant2
  in_D_PI : Subsystem  mask{KP_=KpId_VSC_A, KI_=KiId_VSC_A, Upper_limit=inf, Lower_limit=-inf, Upper_saturation_limit=inf, Lower_saturation_limit=-inf, integrator_init=Md_A_0}
      mask prompts: KP_ "比例系数P"; KI_ "积分系数I"; Upper_limit "限幅上限"; Lower_limit "限幅下限"; Upper_saturation_limit "积分饱和上限"; Lower_saturation_limit "积分饱和下限"; integrator_init "积分初始值"
      mask DialogControl Container4 Prompt: 控制参数
      mask DialogControl Container5 Prompt: 初始值
      mask Display: disp('PI')
  in_Q_PI : Subsystem  mask{KP_=KpIq_VSC_A, KI_=KiIq_VSC_A, Upper_limit=inf, Lower_limit=-inf, Upper_saturation_limit=inf, Lower_saturation_limit=-inf, integrator_init=Mq_A_0}
      mask prompts: KP_ "比例系数P"; KI_ "积分系数I"; Upper_limit "限幅上限"; Lower_limit "限幅下限"; Upper_saturation_limit "积分饱和上限"; Lower_saturation_limit "积分饱和下限"; integrator_init "积分初始值"
      mask DialogControl Container4 Prompt: 控制参数
      mask DialogControl Container5 Prompt: 初始值
      mask Display: disp('PI')
  ucx : Outport
  ucy : Outport  Port=2
  wires:
  Magnitude-Angle to Complex/1 -> Complex to Real-Imag1/1
  Add/1 -> Real-Imag to Complex/2
  Add2/1 -> Real-Imag to Complex/1
  delta/1 -> Add6/2
  Add6/1 -> Magnitude-Angle to Complex/2
  Complex to Magnitude-Angle/2 -> Add6/1
  Sum9/1 -> in_D_PI/1(In1)
  K5/1 -> Add3/1
  [usd] -> Add3/2
  Add3/1 -> Add2/2
  in_D_PI/1(Out1) -> Add2/1
  Constant/1 -> Product4/2
  [isq] -> Product4/1
  [isd] -> Sum9/2
  Product4/1 -> K5/1
  Demux1/1 -> [isd]
  Demux/1 -> [usd]
  Demux1/2 -> [isq]
  Demux/2 -> [usq]
  isdq/1 -> Demux1/1
  usdq/1 -> Demux/1
  [usq] -> Add4/2
  K6/1 -> Add4/1
  in_Q_PI/1(Out1) -> Add/1
  Sum23/1 -> in_Q_PI/1(In1)
  [isd] -> Product1/1
  [isq] -> Sum23/2
  Product1/1 -> K6/1
  Constant4/1 -> Product1/2
  Add4/1 -> Add/2
  Real-Imag to Complex/1 -> Complex to Magnitude-Angle/1
  Complex to Magnitude-Angle/1 -> Magnitude-Angle to Complex/1
  Complex to Real-Imag1/1 -> ucx/1
  Complex to Real-Imag1/2 -> ucy/1
  [usd] -> Scope1/1, control_AC_voltage/1(usd)
  control_AC_voltage/1(isdref) -> Scope7/1, Sum9/1
  [isq] -> Product5/2
  Product5/1 -> Add7/2
  [usd] -> Product5/1
  [isd] -> Product6/2
  Product6/1 -> Add7/1
  [usq] -> Product6/1
  Gain/1 -> Sum/2
  control_AC_voltage1/1(isqref) -> Sum23/1
  [usq] -> Scope2/1, control_AC_voltage1/1(usq)
  Constant2/1 -> control_AC_voltage1/2(usqref)
  Add7/1 -> Scope/1, Gain1/1
  Sum2/1 -> Gain/1
  Constant3/1 -> Sum2/2
  Gain1/1 -> Sum2/1
  Sum/1 -> control_AC_voltage/2(usdref)
  Constant1/1 -> Sum/1

== system M10B39/Genrators/ES3/in_D_PI ==
  In1 : Inport
  Ki : Gain  Gain=KI_  SaturateOnIntegerOverflow=on  OutDataTypeStr=Inherit: Same as input  ParamDataTypeStr=Inherit: Same as input
  Kp : Gain  Gain=KP_  SaturateOnIntegerOverflow=on  OutDataTypeStr=Inherit: Same as input  ParamDataTypeStr=Inherit: Same as input
  Saturation2 : Saturate  UpperLimit=Upper_limit  LowerLimit=Lower_limit
  Sum12 : Sum  SaturateOnIntegerOverflow=on
  integrator : Integrator  InitialCondition=integrator_init  LimitOutput=on  UpperSaturationLimit=Upper_saturation_limit  LowerSaturationLimit=Lower_saturation_limit
  Out1 : Outport
  wires:
  In1/1 -> Ki/1, Kp/1
  Kp/1 -> Sum12/2
  Ki/1 -> integrator/1
  integrator/1 -> Sum12/1
  Saturation2/1 -> Out1/1
  Sum12/1 -> Saturation2/1

== system M10B39/Genrators/ES3/output ==
  is_xy : Inport
  Pe : Inport  Port=2
  Brecx : Constant  Value=0
  Brecy : Constant  Value=0
  Bus Creator : BusCreator  Inputs=4
  Constant : Constant
  Gain : Gain  Gain=SvscB./SgridB
  Gain1 : Gain  Gain=-1
  Gain2 : Gain  Gain=-1
  Gain6 : Gain
  Grecx : Constant  Value=0
  Grecy : Constant  Value=0
  Mux3 : Mux
  Sum : Sum  Inputs=|++
  m : Outport
  isxy : Outport  Port=2
  GBxy : Outport  Port=3
  wires:
  Bus Creator/1 -> m/1
  Gain6/1 -> GBxy/1, Bus Creator/4  "GBxy"
  Mux3/1 -> Gain6/1
  Grecx/1 -> Mux3/1
  Brecx/1 -> Mux3/3
  Grecy/1 -> Mux3/2
  Brecy/1 -> Mux3/4
  Gain1/1 -> isxy/1, Bus Creator/1  "is_xy"
  Gain2/1 -> Bus Creator/2  "Pe"
  Gain/1 -> Gain1/1  "is_xy"
  Pe/1 -> Gain2/1  "Pe"
  Constant/1 -> Sum/2
  [WreES3] -> Sum/1  "Pe"
  Sum/1 -> Bus Creator/3  "w"
  is_xy/1 -> Gain/1

== system M10B39/Genrators/ES3/xy->dq ==
  Ixy : Inport
  Theta : Inport  Port=2
  Complex to Magnitude-Angle : ComplexToMagnitudeAngle
  Complex to Real-Imag : ComplexToRealImag
  Demux1 : Demux  Outputs=2
      settings: DisplayOption=none
  Magnitude-Angle to Complex : MagnitudeAngleToComplex
  Mux : Mux  Inputs=2
  Real-Imag to Complex : RealImagToComplex
  Scope : Scope
      settings: ActiveDisplayYMinimum=3.11918  ActiveDisplayYMaximum=3.16079
  Scope1 : Scope
      settings: ActiveDisplayYMinimum=2.59405  ActiveDisplayYMaximum=3.13201  DataLoggingVariableName=ScopeData3
  Sum1 : Sum  Inputs=|+-  SaturateOnIntegerOverflow=on
  Idq : Outport
  wires:
  Complex to Magnitude-Angle/1 -> Magnitude-Angle to Complex/1
  Theta/1 -> Sum1/2
  Complex to Magnitude-Angle/2 -> Sum1/1, Scope1/1
  Demux1/1 -> Real-Imag to Complex/1
  Complex to Real-Imag/2 -> Mux/2  "Iq"
  Mux/1 -> Idq/1
  Complex to Real-Imag/1 -> Mux/1  "Id"
  Magnitude-Angle to Complex/1 -> Complex to Real-Imag/1
  Sum1/1 -> Magnitude-Angle to Complex/2, Scope/1
  Demux1/2 -> Real-Imag to Complex/2
  Real-Imag to Complex/1 -> Complex to Magnitude-Angle/1
  Ixy/1 -> Demux1/1

== system M10B39/Genrators/Generator1/Excitation System ST1A1 ==
  note: Ef
  Upss : Inport
  Trip : Inport  Port=2
  Vg : Inport  Port=3
  Constant1 : Constant  Value=0
  Ef1 : Integrator  InitialCondition=Ef10
  K : Gain  Gain=1/Tb  SaturateOnIntegerOverflow=on  OutDataTypeStr=Inherit: Same as input  ParamDataTypeStr=Inherit: Same as input
  KA : Gain  Gain=Ka  SaturateOnIntegerOverflow=on  OutDataTypeStr=Inherit: Same as input  ParamDataTypeStr=Inherit: Same as input
  KA1 : Gain  Gain=Tc/Tb  SaturateOnIntegerOverflow=on  OutDataTypeStr=Inherit: Same as input  ParamDataTypeStr=Inherit: Same as input
  KA2 : Gain  Gain=(1/Tb)*(1-Tc/Tb)  SaturateOnIntegerOverflow=on  OutDataTypeStr=Inherit: Same as input  ParamDataTypeStr=Inherit: Same as input
  Saturation : Saturate  UpperLimit=Efmax  LowerLimit=Efmin
  Sum : Sum  Inputs=|++  SaturateOnIntegerOverflow=on
  Sum1 : Sum  Inputs=|+-  SaturateOnIntegerOverflow=on
  Sum4 : Sum  Inputs=|+-+  SaturateOnIntegerOverflow=on
  Switch2 : Switch  Criteria=u2 ~= 0  Threshold=0.5  InputSameDT=off
  Switch3 : Switch  Criteria=u2 ~= 0  Threshold=0.5  InputSameDT=off
  Vref : Constant  Value=Vref
  Ef : Outport
  wires:
  Trip/1 -> Switch3/2, Switch2/2
  Constant1/1 -> Switch3/1, Switch2/1
  Switch3/1 -> KA2/1, K/1
  Ef1/1 -> Switch3/3
  Switch2/1 -> Ef1/1
  Sum1/1 -> Switch2/3
  KA/1 -> KA1/1, Sum1/1
  Upss/1 -> Sum4/3
  Saturation/1 -> Ef/1
  Vg/1 -> Sum4/2
  Sum4/1 -> KA/1
  Vref/1 -> Sum4/1
  Sum/1 -> Saturation/1
  K/1 -> Sum1/2
  KA1/1 -> Sum/2
  KA2/1 -> Sum/1

== system M10B39/Genrators/Generator1/Governor ==
  w : Inport
  Trip : Inport  Port=2
  CT : Constant  Value=0
  Constant : Constant  Value=0
  Gain : Gain  Gain=a_G  SaturateOnIntegerOverflow=on  OutDataTypeStr=Inherit: Same as input  ParamDataTypeStr=Inherit: Same as input
  Saturation : Saturate  UpperLimit=dPmax  LowerLimit=dPmin
  Sum1 : Sum  Inputs=|++  SaturateOnIntegerOverflow=on
  Sum3 : Sum  Inputs=|+-  SaturateOnIntegerOverflow=on
  Switch : Switch  Threshold=0.5  InputSameDT=off
  Switch1 : Switch  Criteria=u2 ~= 0  Threshold=0.5  InputSameDT=off
  Transfer Fcn1 : TransferFcn  Numerator=[b_G]  Denominator=[Tg_G 1]
  w0 : Gain  Gain=wB  SaturateOnIntegerOverflow=on  OutDataTypeStr=Inherit: Same as input  ParamDataTypeStr=Inherit: Same as input
  w1 : Constant  Value=S_Gov
  wref : Constant
  dPm : Outport
  wires:
  Gain/1 -> Sum1/1
  w1/1 -> Switch/2
  CT/1 -> Switch/3
  Sum3/1 -> w0/1
  Sum1/1 -> Saturation/1
  Saturation/1 -> Switch/1
  wref/1 -> Sum3/1
  w0/1 -> Gain/1, Transfer Fcn1/1
  Transfer Fcn1/1 -> Sum1/2
  w/1 -> Sum3/2
  Constant/1 -> Switch1/1
  Switch/1 -> Switch1/3
  Trip/1 -> Switch1/2
  Switch1/1 -> dPm/1

== system M10B39/Genrators/Generator1/Machine Equations  ==
  note: Iqg
  note: Idg
  note: 接口
  delta : Inport
  Vgxy : Inport  Port=2
  Ef : Inport  Port=3
  Trip : Inport  Port=4
  Demux : Demux  Outputs=2
  Demux1 : Demux  Outputs=2
  Fcn1 : Fcn  Expr=u(1)*u(3)+u(2)*u(4)
  Fcn2 : Fcn  Expr=(u(3)-u(2))/Xd1
  Fcn3 : Fcn  Expr=(u(1)-u(4))/Xq1
  Fcn4 : Fcn  Expr=u(2)*u(3)-u(1)*u(4)
  Fcn6 : Fcn  Expr=sqrt(u(1)^2+u(2)^2)
  Interface : Subsystem
  Mux1 : Mux  Inputs=2
  Mux2 : Mux  Inputs=2
  Mux3 : Mux  Inputs=2
  Qe : Scope
      settings: TimeSpan=10  ActiveDisplayYMinimum=0.15  ActiveDisplayYMaximum=0.65
  Scope{,1..3} (4 alike) : Scope
      Scope settings: ActiveDisplayYMinimum=6.90941  ActiveDisplayYMaximum=6.93032
      Scope1 settings: ActiveDisplayYMinimum=0.73198  ActiveDisplayYMaximum=0.74189  DataLoggingVariableName=ScopeData2
      Scope2 settings: ActiveDisplayYMinimum=0.70724  ActiveDisplayYMaximum=0.71179  DataLoggingVariableName=ScopeData3
      Scope3 settings: ActiveDisplayYMinimum=3.59596  ActiveDisplayYMaximum=3.95434  DataLoggingVariableName=ScopeData4
  Transient Equations : Subsystem
  Pe : Outport
  Igxy1 : Outport  Port=2
  GBxy : Outport  Port=3
  Vg : Outport  Port=4
  wires:
  Trip/1 -> Transient Equations/3(Trip)
  Demux1/2 -> Scope3/1
  Demux/2 -> Scope2/1
  Demux1/1 -> Scope/1
  Demux/1 -> Scope1/1
  Transient Equations/1(Eqd') -> Interface/3(Eqd''), Mux1/2
  Interface/3(GBxy) -> GBxy/1
  Interface/2(Igxy1) -> Igxy1/1
  Vgxy/1 -> Interface/2(Vgxy)
  delta/1 -> Interface/1(delta)
  Fcn4/1 -> Qe/1
  Fcn6/1 -> Vg/1
  Fcn1/1 -> Pe/1
  Ef/1 -> Transient Equations/2(Ef)
  Mux2/1 -> Fcn4/1, Fcn1/1
  Mux1/1 -> Fcn3/1, Fcn2/1
  Interface/1(Vdqg) -> Mux1/1, Fcn6/1, Mux2/1, Demux/1
  Mux3/1 -> Mux2/2, Demux1/1, Transient Equations/1(Idqg)
  Fcn2/1 -> Mux3/1
  Fcn3/1 -> Mux3/2

== system M10B39/Genrators/Generator1/Mechanical DE ==
  Pe : Inport
  dPm : Inport  Port=2
  Trip : Inport  Port=3
  Constant1 : Constant  Value=0
  Constant2 : Constant  Value=0
  Gain : Gain  Gain=wB  SaturateOnIntegerOverflow=on  OutDataTypeStr=Inherit: Same as input  ParamDataTypeStr=Inherit: Same as input
  Gain1 : Gain  Gain=1/H  SaturateOnIntegerOverflow=on  OutDataTypeStr=Inherit: Same as input  ParamDataTypeStr=Inherit: Same as input
  Gain2 : Gain  Gain=D  SaturateOnIntegerOverflow=on  OutDataTypeStr=Inherit: Same as input  ParamDataTypeStr=Inherit: Same as input
  Gain5 : Gain  Gain=180/pi  SaturateOnIntegerOverflow=on  OutDataTypeStr=Inherit: Same as input  ParamDataTypeStr=Inherit: Same as input
  Int1 : Integrator  InitialCondition=delta0
  Int2 : Integrator  InitialCondition=w0
  Pm : Constant  Value=Pm0
  Scope2 : Scope
      settings: TimeSpan=10  ActiveDisplayYMinimum=-0.4  ActiveDisplayYMaximum=1.4  DataLoggingVariableName=ScopeData5
  Scope4 : Scope
      settings: TimeSpan=10  ActiveDisplayYMinimum=0.99999999999991518  ActiveDisplayYMaximum=1.0000000000005032  DataLoggingVariableName=ScopeData6
  Scope8 : Scope
      settings: TimeSpan=10  ActiveDisplayYMinimum=-0.4  ActiveDisplayYMaximum=1.4  DataLoggingVariableName=ScopeData11
  Sum2 : Sum  Inputs=-+-+  SaturateOnIntegerOverflow=on
  Sum3 : Sum  Inputs=|+-  SaturateOnIntegerOverflow=on
  Switch{1..4} (4 alike) : Switch  Criteria=u2 ~= 0  Threshold=0.5  InputSameDT=off
  w0 : Constant
  delta : Outport
  w : Outport  Port=2
  wires:
  [Trip] -> Switch3/2, Switch2/2
  Constant1/1 -> Switch3/1, Switch2/1
  Switch3/1 -> Scope4/1, Sum3/1, w/1
  Int2/1 -> Switch3/3
  Switch2/1 -> Int2/1
  Gain1/1 -> Switch2/3
  Trip/1 -> [Trip]
  [Trip] -> Switch1/2, Switch4/2
  Constant2/1 -> Switch4/1, Switch1/1
  Switch4/1 -> delta/1, Scope2/1, Gain5/1
  Int1/1 -> Switch4/3
  Switch1/1 -> Int1/1
  Gain/1 -> Switch1/3
  Gain5/1 -> Scope8/1
  w0/1 -> Sum3/2
  Sum3/1 -> Gain2/1, Gain/1
  Pm/1 -> Sum2/2
  Gain2/1 -> Sum2/1
  Sum2/1 -> Gain1/1
  Pe/1 -> Sum2/3
  dPm/1 -> Sum2/4

== system M10B39/Genrators/Generator1/Output ==
  Igxy1in : Inport
  GBxyin : Inport  Port=2
  deltain : Inport  Port=3
  Pein : Inport  Port=4
  fin : Inport  Port=5
  Vg : Inport  Port=6
  Bus Creator : BusCreator  Inputs=6
  m : Outport
  Igxy1 : Outport  Port=2
  GBxy : Outport  Port=3
  wires:
  Vg/1 -> Bus Creator/6  "Vg"
  fin/1 -> Bus Creator/5  "f"
  Pein/1 -> Bus Creator/4  "Pe"
  deltain/1 -> Bus Creator/3  "delta"
  GBxyin/1 -> Bus Creator/2, GBxy/1  "GBxy"
  Igxy1in/1 -> Bus Creator/1, Igxy1/1  "Igxy1"
  Bus Creator/1 -> m/1

== system M10B39/Genrators/Generator1/PSS1 ==
  w : Inport
  Trip : Inport  Port=2
  CT : Constant  Value=0
  Constant : Constant  Value=0
  Gain : Gain  Gain=Kpss  SaturateOnIntegerOverflow=on  OutDataTypeStr=Inherit: Same as input  ParamDataTypeStr=Inherit: Same as input
  Saturation : Saturate  UpperLimit=Upmax  LowerLimit=Upmin
  Sum3 : Sum  Inputs=|+-  SaturateOnIntegerOverflow=on
  Switch : Switch  Threshold=0.5  InputSameDT=off
  Switch1 : Switch  Threshold=0.5  InputSameDT=off
  Transfer Fcn : TransferFcn  Numerator=[Tw_P 0]  Denominator=[Tw_P 1]
  Transfer Fcn1 : TransferFcn  Numerator=[T1_P 1]  Denominator=[T2_P 1]
  Transfer Fcn2 : TransferFcn  Numerator=[T3_P 1]  Denominator=[T4_P 1]
  w0 : Constant
  w1 : Constant  Value=S_PSS
  Upss : Outport
  wires:
  Constant/1 -> Switch1/1
  Trip/1 -> Switch1/2
  Switch1/1 -> Upss/1
  Switch/1 -> Switch1/3
  Transfer Fcn/1 -> Transfer Fcn1/1
  Gain/1 -> Transfer Fcn/1
  w1/1 -> Switch/2
  CT/1 -> Switch/3
  Saturation/1 -> Switch/1
  Sum3/1 -> Gain/1
  Transfer Fcn2/1 -> Saturation/1
  Transfer Fcn1/1 -> Transfer Fcn2/1
  w/1 -> Sum3/1
  w0/1 -> Sum3/2

== system M10B39/Genrators/Wind Generator - DFIG1/Asynchronous Machine Equations  ==
  note: Vsdq
  s / ω_B : Inport
  Vgxy : Inport  Port=2
  Vrxy : Inport  Port=3
  "Trip " : Inport  Port=4
  3th order Transient Equations : Subsystem
  Add : Sum  Inputs=+-
  Constant : Constant  Value=Za
  Constant1 : Constant  Value=0
  Fcn6 : Fcn  Expr=sqrt(u(1)^2+u(2)^2)
  Gain2 : Gain  Gain=NPf
  Interface : Subsystem
  Multiply : Product  Multiplication=Matrix(*)
  Mux2 : Mux  Inputs=2
  Mux4 : Mux  Inputs=2
  Ps_ : Fcn  Expr=u(1)*u(3)+u(2)*u(4)
  Qs_ : Fcn  Expr=u(2)*u(3)-u(1)*u(4)
  Scope : Scope
      settings: ActiveDisplayYMinimum=-0.69793  ActiveDisplayYMaximum=9.95802
  Scope1 : Scope
      settings: ActiveDisplayYMinimum=0.89985  ActiveDisplayYMaximum=1.09985
  Selector : Selector  InputPortWidth=2  IndexOptions=Index vector (dialog)  Indices=[2 1]  OutputSizes=1
  Te_ : Fcn  Expr=u(2)*u(3)+u(1)*u(4)
  Te : Outport
  Ps : Outport  Port=2
  Qs : Outport  Port=3
  Irxy : Outport  Port=4
  Exy : Outport  Port=5
  Isxy1 : Outport  Port=6
  GBxy : Outport  Port=7
  wires:
  "Trip "/1 -> 3th order Transient Equations/4(Trip)
  3th order Transient Equations/1(Irxy) -> Irxy/1
  Qs_/1 -> Qs/1, Scope/1
  Constant1/1 -> Interface/1(delta)
  Gain2/1 -> Te/1
  Vgxy/1 -> Add/1, Fcn6/1, Mux2/1
  Add/1 -> Multiply/2
  Constant/1 -> Multiply/1
  Selector/1 -> Exy/1, Add/2
  Te_/1 -> Gain2/1
  Mux4/1 -> Te_/1
  s / ω_B/1 -> 3th order Transient Equations/3(s / ω_B)
  Ps_/1 -> Ps/1
  Interface/1(Igxy1) -> Isxy1/1
  Interface/2(GBxy) -> GBxy/1
  Mux2/1 -> Qs_/1, Ps_/1
  Vrxy/1 -> 3th order Transient Equations/2(Vrxy)
  Multiply/1 -> 3th order Transient Equations/1(Isxy), Mux4/1, Mux2/2
  Fcn6/1 -> Scope1/1
  3th order Transient Equations/2(Eyx) -> Mux4/2, Selector/1, Interface/2(Eqd)

== system M10B39/Genrators/Wind Generator - DFIG1/Converter function ==
  Vsxy : Inport
  Vcxy : Inport  Port=2
  Trip : Inport  Port=3
  Change_choke : Gain  Gain=[1 -1]  SaturateOnIntegerOverflow=on  OutDataTypeStr=Inherit: Same as input  ParamDataTypeStr=Inherit: Same as input
  Constant2 : Constant  Value=0
  GSC_Idq : Integrator  InitialCondition=[Icx0 Icy0]
  L_choke : Gain  Gain=Lg  SaturateOnIntegerOverflow=on  OutDataTypeStr=Inherit: Same as input  ParamDataTypeStr=Inherit: Same as input
  R_choke : Gain  Gain=Rg  SaturateOnIntegerOverflow=on  OutDataTypeStr=Inherit: Same as input  ParamDataTypeStr=Inherit: Same as input
  Selector : Selector  InputPortWidth=2  IndexOptions=Index vector (dialog)  Indices=[2 1]  OutputSizes=1
  Sum : Sum  Inputs=+--+  SaturateOnIntegerOverflow=on
  Switch1 : Switch  Criteria=u2 ~= 0  Threshold=0.5  InputSameDT=off
  Switch4 : Switch  Criteria=u2 ~= 0  Threshold=0.5  InputSameDT=off
  W/L : Gain  Gain=wB / Lg  SaturateOnIntegerOverflow=on  OutDataTypeStr=Inherit: Same as input  ParamDataTypeStr=Inherit: Same as input
  Ixy_gsc : Outport
  wires:
  Switch4/1 -> Ixy_gsc/1, R_choke/1, Selector/1
  GSC_Idq/1 -> Switch4/3
  Switch1/1 -> GSC_Idq/1
  W/L/1 -> Switch1/3
  Constant2/1 -> Switch4/1, Switch1/1
  Trip/1 -> Switch1/2, Switch4/2
  Vcxy/1 -> Sum/2
  Change_choke/1 -> Sum/4
  Sum/1 -> W/L/1
  R_choke/1 -> Sum/3
  Vsxy/1 -> Sum/1
  Selector/1 -> L_choke/1
  L_choke/1 -> Change_choke/1

== system M10B39/Genrators/Wind Generator - DFIG1/DC Bus model ==
  note: Pdc = Pr_gsc - Pr_rsc
  Pr_gsc : Inport
  Pr_rsc : Inport  Port=2
  Product2 : Product  Inputs=*/  InputSameDT=on  SaturateOnIntegerOverflow=on  OutDataTypeStr=Inherit: Same as first input
  Sum2 : Sum  Inputs=+-  InputSameDT=on  SaturateOnIntegerOverflow=on  OutDataTypeStr=Inherit: Same as first input
  Udc : Integrator  InitialCondition=Vdc0  LowerSaturationLimit=1e-6  ZeroCross=off
  deg->rad1 : Gain  Gain=1/C_w  SaturateOnIntegerOverflow=on  OutDataTypeStr=Inherit: Same as input  ParamDataTypeStr=Inherit: Same as input
  deg->rad2 : Gain  Gain=wB  SaturateOnIntegerOverflow=on  OutDataTypeStr=Inherit: Same as input  ParamDataTypeStr=Inherit: Same as input
  Vdc : Outport
  wires:
  deg->rad2/1 -> deg->rad1/1
  Sum2/1 -> Product2/1
  deg->rad1/1 -> Udc/1
  Pr_gsc/1 -> Sum2/1
  Product2/1 -> deg->rad2/1  "Idc"
  Udc/1 -> Product2/2, Vdc/1  "Vdc"
  Pr_rsc/1 -> Sum2/2

== system M10B39/Genrators/Wind Generator - DFIG1/Grid Side Converter and control ==
  note: K为系数，p/i为系数的名字，DC/Id/Iq为控制的量，g为GSC，w为wind，与直流电网的VSC参数区分开来
  Vdc : Inport
  Vsdq : Inport  Port=2
  Icdq : Inport  Port=3
  Enable : EnablePort
  Add : Sum  Inputs=|+-
  Add{1,3,5,7,11} (5 alike) : Sum
  Add10 : Sum  Commented=on
  Add2 : Sum  Inputs=|+-
  Add4 : Sum  Inputs=|-+
  Add6 : Sum  Inputs=|+-
  Add8 : Sum  Inputs=|-+
  Add9 : Sum  Inputs=-+
  Constant : Constant  Value=Vdc_w
  Constant1 : Constant  Value=Icq_ref
  Constant2 : Constant
  Demux : Demux  Outputs=2
  Demux1 : Demux  Outputs=2
  From12 : From  Commented=on  GotoTag=Icd
  From13 : From  Commented=on  GotoTag=Icq
  From14 : From  Commented=on  GotoTag=Ucd
  From15 : From  Commented=on  GotoTag=Ucq
  Gain : Gain  Gain=KpDC_gw
  Gain1 : Gain  Gain=KiDC_gw
  Gain2 : Gain  Gain=KpId_gw
  Gain3 : Gain  Gain=KiId_gw
  Gain4 : Gain  Gain=Lg
  Gain5 : Gain  Gain=KpIq_gw
  Gain6 : Gain  Gain=KiIq_gw
  Gain7 : Gain  Gain=Lg
  KiDC_gw : Integrator  InitialCondition=Icd_ref
  KiId_gw : Integrator
  KiIq_gw : Integrator
  Multiply{,1,4..5} (4 alike) : Product
  Multiply2 : Product  Commented=on
  Multiply3 : Product  Commented=on
  Mux : Mux  Inputs=2
  Scope1 : Scope
      settings: ActiveDisplayYMinimum=0.114016671  ActiveDisplayYMaximum=0.114016689  DataLoggingVariableName=ScopeData4
  Scope3 : Scope
      settings: ActiveDisplayYMinimum=-1.4E-17  ActiveDisplayYMaximum=9E-18  DataLoggingVariableName=ScopeData11
  Scope4 : Scope
      settings: ActiveDisplayYMinimum=-0.04026  ActiveDisplayYMaximum=0.20394  DataLoggingVariableName=ScopeData12
  Pr_gsc : Outport
  ucdq : Outport  Port=2
  wires:
  Demux1/2 -> [Icq]
  Icdq/1 -> Demux1/1
  Demux1/1 -> [Icd]
  Mux/1 -> ucdq/1
  Add8/1 -> Mux/2
  Add4/1 -> Mux/1
  Add6/1 -> Gain5/1, Gain6/1, Scope3/1
  Add11/1 -> Pr_gsc/1
  Multiply5/1 -> Add11/2
  Multiply4/1 -> Add11/1
  [Vsd] -> Multiply4/1
  [Vsq] -> Multiply5/1
  [Icd] -> Multiply4/2
  [Icq] -> Multiply5/2
  From14/1 -> Multiply2/1
  From12/1 -> Multiply2/2
  Multiply2/1 -> Add10/1
  From15/1 -> Multiply3/1
  From13/1 -> Multiply3/2
  Multiply3/1 -> Add10/2
  Add9/1 -> Add8/2
  Multiply1/1 -> Gain7/1
  [Icd] -> Multiply1/2
  Gain7/1 -> Add9/1
  [Vsq] -> Add9/2
  [We] -> Multiply1/1
  Gain6/1 -> KiIq_gw/1
  Gain5/1 -> Add7/1
  KiIq_gw/1 -> Add7/2
  Add7/1 -> Add8/1  "Vgq'"
  Constant1/1 -> Add6/1
  [Icq] -> Add6/2
  [Vsd] -> Add5/2
  Demux/1 -> [Vsd]
  Demux/2 -> [Vsq]
  Vsdq/1 -> Demux/1, [Vsdq]
  Add5/1 -> Add4/2
  Gain4/1 -> Add5/1
  [Icq] -> Multiply/2
  Multiply/1 -> Gain4/1
  [We] -> Multiply/1
  Add3/1 -> Add4/1  "Vgd'"
  Gain3/1 -> KiId_gw/1
  KiId_gw/1 -> Add3/2
  Add2/1 -> Gain2/1, Gain3/1, Scope4/1
  Gain2/1 -> Add3/1
  [Icd] -> Add2/2, Scope1/1
  Add1/1 -> Add2/1  "Iref_cd*"
  KiDC_gw/1 -> Add1/2
  Gain1/1 -> KiDC_gw/1
  Gain/1 -> Add1/1
  Add/1 -> Gain/1, Gain1/1
  [Vdc] -> Add/2
  Constant/1 -> Add/1
  Constant2/1 -> [We]
  Vdc/1 -> [Vdc]

== system M10B39/Genrators/Wind Generator - DFIG1/Mechanical DE ==
  note: 这里是电动机惯例，因此发电的时候力矩应该是负的
  note: $\frac{d\omega_r}{dt}=\frac{1}{H}(T_e-T_m)$
      | 电动机惯例
  Te : Inport
  Tm : Inport  Port=2
  AWr : Integrator  InitialCondition=Wr0
  Add : Sum  Inputs=+-
  Constant2 : Constant
  Gain : Gain  Gain=1/H
  Scope : Scope
      settings: ActiveDisplayYMinimum=0.89006  ActiveDisplayYMaximum=0.98946
  Scope2 : Scope
      settings: ActiveDisplayYMinimum=-0.25  ActiveDisplayYMaximum=2.25  DataLoggingVariableName=ScopeData4
  Sum : Sum  Inputs=|-+
  "s " : Outport
  Wr : Outport  Port=2
  wires:
  Sum/1 -> "s "/1
  Tm/1 -> Scope2/1, Add/2
  Add/1 -> Gain/1
  Constant2/1 -> Sum/2
  Gain/1 -> AWr/1
  Te/1 -> Add/1
  AWr/1 -> Sum/1, Wr/1, Scope/1
